simulink model "FullModelAddANN_Final_ANN_revised"  (R2024b)
settings: Solver=ode4  StartTime=0.0  StopTime=40  FixedStep=1e-5  RelTol=1e-3
values from neighbouring files (symbols this model uses):
  Dp = 2.506338228783948e3    (= 2506.33822878)    [FullModelAddANNm_Final.m]    (also in main_opal_ann_control.m)
  Dq = 1.033099625954584    (= 1.03309962595)    [FullModelAddANNm_Final.m]    (also in main_opal_ann_control.m)
  Kp = 0.006383815167581    (= 0.00638381516758)    [FullModelAddANNm_Final.m]    (also in main_opal_ann_control.m)
  Kq = 0.076670166944346    (= 0.0766701669443)    [FullModelAddANNm_Final.m]    (also in main_opal_ann_control.m)
undefined symbols (not defined in the file or in its folder): Filter, Ls, params
libraries: neural x88, spsCurrentMeasurementLib x6, spsParallelRLCBranchLib x6, spsIGBTDiodeLib x6, spsMeanLib x6, spsSeriesRLCBranchLib x6, simulink x4, spsVoltageMeasurementLib x4, spsVariableInductorLib x3, spsVariableResistorLib x3, spsDCVoltageSourceLib x1, spsThreePhaseSourceLib x1
(part 5 of 11)

== system FullModelAddANN_Final_ANN_revised/Feed-Forward Neural Network2/Layer 2/Delays 1 ==
  "p{2}" : Inport  PortDimensions=16
      mask Display: e = 0.06;c1 = [120 230 180]/255;c2 = ([120 230 180]+0)/(256+128);c3 = ([120 230 180]+128)/(256+128);patch([0 1 1 0],[0 0 1 1],c1);patch([0 1 1 1-e 1-e 0+e],[0 0 1 1-e 0+e 0+e],c2);patch([0 0 1 1-e 0+e 0+e],[0 1 1 1-e 1-e 0+e],c3);plot([0 1 1 0 0],[0 0 1 1 0]);
  mux : Mux  Inputs=1
      mask Display: e = 0.06;c1 = [120 150 230]/255;c2 = ([120 150 230]+0)/383;c3 = ([120 150 230]+128)/383;patch([0 1 1 0],[0 0 1 1],c1);patch([0 1 1 1-e 1-e 0+e],[0 0 1 1-e 0+e 0+e],c2);patch([0 0 1 1-e 0+e 0+e],[0 1 1 1-e 1-e 0+e],c3);plot([0 1 1 0 0],[0 0 1 1 0]);disp('Mux')
  "pd{2,1}" : Outport
      mask Display: e = 0.06;c1 = [120 230 180]/255;c2 = ([120 230 180]+0)/(256+128);c3 = ([120 230 180]+128)/(256+128);patch([0 1 1 0],[0 0 1 1],c1);patch([0 1 1 1-e 1-e 0+e],[0 0 1 1-e 0+e 0+e],c2);patch([0 0 1 1-e 0+e 0+e],[0 1 1 1-e 1-e 0+e],c3);plot([0 1 1 0 0],[0 0 1 1 0]);
  wires:
  "p{2}"/1 -> mux/1
  mux/1 -> "pd{2,1}"/1

== system FullModelAddANN_Final_ANN_revised/Feed-Forward Neural Network2/Layer 2/LW{2,1} ==
  "ad{2,1}" : Inport  PortDimensions=16
      mask Display: e = 0.06;c1 = [120 230 180]/255;c2 = ([120 230 180]+0)/(256+128);c3 = ([120 230 180]+128)/(256+128);patch([0 1 1 0],[0 0 1 1],c1);patch([0 1 1 1-e 1-e 0+e],[0 0 1 1-e 0+e 0+e],c2);patch([0 0 1 1-e 0+e 0+e],[0 1 1 1-e 1-e 0+e],c3);plot([0 1 1 0 0],[0 0 1 1 0]);
  "IW{2,1}(1,:)'" : Constant  Value=[0.0619006782895638874020249886598321609199047088623046875;0.1686426640227181028564018561155535280704498291015625;0.52423236288504215796280050199129618704319000244140625;-0.1209574734873513912614129139910801313817501068115234375;0.10374581170755874104383309486365760676562786102294921875;0.4130990285372890813420099220820702612400054931640625;0.061020386022926302593827330156273092143237590789794921875;1.304235337766612712329106216202490031719207763671875;0.173065812923836548353762054830440320074558258056640625;0.1850513487771471010656654243575758300721645355224609375;-0.003234637058241617534048994997419868013821542263031005859375;-0.1648403386263822267832068746429285965859889984130859375;-0.255677464090604822377628124741022475063800811767578125;0.368145708619515676929268011008389294147491455078125;-0.1075705688767357448565320510169840417802333831787109375;-0.01777056305149475601279362990680965594947338104248046875]
      mask Display: e = 0.06;c1 = [120 150 230]/255;c2 = ([120 150 230]+0)/383;c3 = ([120 150 230]+128)/383;patch([0 1 1 0],[0 0 1 1],c1);patch([0 1 1 1-e 1-e 0+e],[0 0 1 1-e 0+e 0+e],c2);patch([0 0 1 1-e 0+e 0+e],[0 1 1 1-e 1-e 0+e],c3);plot([0 1 1 0 0],[0 0 1 1 0]);disp('weights');
  "IW{2,1}(2,:)'" : Constant  Value=[-0.1919079853721659401077914708366733975708484649658203125;0.0769860216421201226655313121227663941681385040283203125;-0.0288224234234223906925276281754122464917600154876708984375;0.11367284231069628430699225418720743618905544281005859375;0.1410010999802841780148554562401841394603252410888671875;-0.112804581549694693531904476913041435182094573974609375;-0.099983026993281043370842553485999815165996551513671875;-0.67737671415215883197191715225926600396633148193359375;1.0726190667598667349835750428610481321811676025390625;-0.298931860532267223984348447629599831998348236083984375;0.0884455568850744111575323813667637296020984649658203125;-0.0079188047282774780277758708280089194886386394500732421875;-0.08177686161481258209082767507425160147249698638916015625;0.0879225019016239561775449828928685747087001800537109375;0.14099923701365491002235330597613938152790069580078125;0.26765837325222896492249446964706294238567352294921875]
      mask Display: e = 0.06;c1 = [120 150 230]/255;c2 = ([120 150 230]+0)/383;c3 = ([120 150 230]+128)/383;patch([0 1 1 0],[0 0 1 1],c1);patch([0 1 1 1-e 1-e 0+e],[0 0 1 1-e 0+e 0+e],c2);patch([0 0 1 1-e 0+e 0+e],[0 1 1 1-e 1-e 0+e],c3);plot([0 1 1 0 0],[0 0 1 1 0]);disp('weights');
  Mux : Mux  Inputs=2
      mask Display: e = 0.06;c1 = [120 150 230]/255;c2 = ([120 150 230]+0)/383;c3 = ([120 150 230]+128)/383;patch([0 1 1 0],[0 0 1 1],c1);patch([0 1 1 1-e 1-e 0+e],[0 0 1 1-e 0+e 0+e],c2);patch([0 0 1 1-e 0+e 0+e],[0 1 1 1-e 1-e 0+e],c3);plot([0 1 1 0 0],[0 0 1 1 0]);disp('Mux');
  dotprod1 : neural/Weight Functions/dotprod
  dotprod2 : neural/Weight Functions/dotprod
  "lz{2,1}" : Outport
      mask Display: e = 0.06;c1 = [120 230 180]/255;c2 = ([120 230 180]+0)/(256+128);c3 = ([120 230 180]+128)/(256+128);patch([0 1 1 0],[0 0 1 1],c1);patch([0 1 1 1-e 1-e 0+e],[0 0 1 1-e 0+e 0+e],c2);patch([0 0 1 1-e 0+e 0+e],[0 1 1 1-e 1-e 0+e],c3);plot([0 1 1 0 0],[0 0 1 1 0]);
  wires:
  "IW{2,1}(1,:)'"/1 -> dotprod1/1
  "ad{2,1}"/1 -> dotprod1/2, dotprod2/2
  dotprod1/1 -> Mux/1
  "IW{2,1}(2,:)'"/1 -> dotprod2/1
  dotprod2/1 -> Mux/2
  Mux/1 -> "lz{2,1}"/1

== system FullModelAddANN_Final_ANN_revised/Feed-Forward Neural Network_Full/Layer 1/Delays 1 ==
  "p{1}" : Inport  PortDimensions=200
      mask Display: e = 0.06;c1 = [120 230 180]/255;c2 = ([120 230 180]+0)/(256+128);c3 = ([120 230 180]+128)/(256+128);patch([0 1 1 0],[0 0 1 1],c1);patch([0 1 1 1-e 1-e 0+e],[0 0 1 1-e 0+e 0+e],c2);patch([0 0 1 1-e 0+e 0+e],[0 1 1 1-e 1-e 0+e],c3);plot([0 1 1 0 0],[0 0 1 1 0]);
  mux : Mux  Inputs=1
      mask Display: e = 0.06;c1 = [120 150 230]/255;c2 = ([120 150 230]+0)/383;c3 = ([120 150 230]+128)/383;patch([0 1 1 0],[0 0 1 1],c1);patch([0 1 1 1-e 1-e 0+e],[0 0 1 1-e 0+e 0+e],c2);patch([0 0 1 1-e 0+e 0+e],[0 1 1 1-e 1-e 0+e],c3);plot([0 1 1 0 0],[0 0 1 1 0]);disp('Mux')
  "pd{1,1}" : Outport
      mask Display: e = 0.06;c1 = [120 230 180]/255;c2 = ([120 230 180]+0)/(256+128);c3 = ([120 230 180]+128)/(256+128);patch([0 1 1 0],[0 0 1 1],c1);patch([0 1 1 1-e 1-e 0+e],[0 0 1 1-e 0+e 0+e],c2);patch([0 0 1 1-e 0+e 0+e],[0 1 1 1-e 1-e 0+e],c3);plot([0 1 1 0 0],[0 0 1 1 0]);
  wires:
  "p{1}"/1 -> mux/1
  mux/1 -> "pd{1,1}"/1
